simulink model "PSO_thuc_nghiem"  (R2021a)
settings: Solver=VariableStepAuto  StartTime=0.0  StopTime=10  RelTol=1e-3
InitFcn:
  | mc=0.5;
  | g=9.81;
  | n1=5;n2=1;
  | 
  | L2=0.5;
  | m1=2;
  | m2=mc;
  | m=5;
  | %Bo input shaping
  | alpha = (1/L1 + 1/L2)*(m1+m2)/m1;
  | beta = (((m1+m2)/m1)^2)*((1/L1 + 1/L2)^2) - 4*(m1+m2)/(m1*L1*L2);
  | w1 = sqrt(g*(alpha - sqrt(beta))/2);
  | w2 = sqrt(g*(alpha + sqrt(beta))/2);
  | damping_ratio = 0;
  | wd1 = w1*sqrt(1-damping_ratio^2);
  | wd2 = w2*sqrt(1-damping_ratio^2);
  | k = exp(damping_ratio*pi/sqrt(1-damping_ratio^2));
  | 
  | %ETM4_1
  | m_etm4_1 = 0.1;
  | I_etm4_1 = (1+m_etm4_1)*k*k/(k^2 + (1+m_etm4_1)*(k^(4/3)+k^(2/3)) + m_etm4_1);
  | A1_etm4_1 = I_etm4_1/(1+m_etm4_1);
  | A2_etm4_1 = I_etm4_1/(k^(2/3));
  | A3_etm4_1 = I_etm4_1/(k^(4/3));
  | A4_etm4_1 = m_etm4_1*I_etm4_1/((1+m_etm4_1)*(k^2));
  | t1_etm4_1 = (2*pi/3)/wd1;
  | t2_etm4_1 = (4*pi/3)/wd1;
  | t3_etm4_1 = 2*pi/wd1;
  | %ETM4_2
  | m_etm4_2 = 0.1;
  | I_etm4_2 = (1+m_etm4_2)*k*k/(k^2 + (1+m_etm4_2)*(k^(4/3)+k^(2/3)) + m_etm4_2);
  | A1_etm4_2 = I_etm4_2/(1+m_etm4_2);
  | A2_etm4_2 = I_etm4_2/(k^(2/3));
  | A3_etm4_2 = I_etm4_2/(k^(4/3));
  | A4_etm4_2 = m_etm4_2*I_etm4_2/((1+m_etm4_2)*(k^2));
  | t1_etm4_2 = (2*pi/3)/wd2;
  | t2_etm4_2 = (4*pi/3)/wd2;
  | t3_etm4_2 = 2*pi/wd2;
values from neighbouring files (symbols this model uses):
  l_ini = L    [PSO_ZVD.m]
  particle = repmat(empty_particle, nPop, 1)    [PSO16_12.m]    (also in PSO_ZVD.m)
undefined symbols (not defined in the file or in its folder): b0, b1, i, Kd, Kd1, Kp, Kp1, l, l1, l11, l2, l21, l3, l31, l_ref, li, M2, x_ref, xi
libraries: neural x70, simulink_extras x11, simulink x5
(part 21 of 25)

== matlab function PSO_thuc_nghiem/non linear model/con lắc đôi2/MATLAB Function ==
  data: z1 input; z2 input; z3 input; z4 input; z5 input; z6 input; z7 input; z8 input; d1z1 output; d1z2 output; d1z3 output; d1z4 output; d1z5 output; d1z6 output; d1z7 output; d1z8 output; ux input; ul input
function [d1z1,d1z2,d1z3,d1z4,d1z5,d1z6,d1z7,d1z8] = fcn(z1,z2, z3, z4, z5, z6, z7, z8, ux, ul)

m=20; m1=5; m2=1; l2= 0.2; g= 9.8;

d1z1=z2;
d1z2 =(m1*ul*sin(z5) - m2*ux - m1*ux + m2*ul*sin(z5) + m2*ux*cos(z5 - z7)^2 + m2*ux*sin(z5 - z7)^2 - m2*ul*sin(z5 - z7)*cos(z7) - g*m2^2*cos(z7)*sin(z7) - l2*m2^2*z8^2*sin(z7) - m2*ul*cos(z5 - z7)^2*sin(z5) + g*m2^2*cos(z5 - z7)*sin(z5 - z7)*cos(z5)^2 - g*m2^2*cos(z5 - z7)*sin(z5 - z7)*sin(z5)^2 + m2*ul*cos(z5 - z7)*sin(z5 - z7)*cos(z5) - g*m1*m2*cos(z7)*sin(z7) - l2*m1*m2*z8^2*sin(z7) + g*m2^2*cos(z5 - z7)*cos(z5)*sin(z7) + g*m2^2*cos(z5 - z7)*cos(z7)*sin(z5) - g*m2^2*sin(z5 - z7)*cos(z5)*cos(z7) + l2*m2^2*z8^2*cos(z5 - z7)*sin(z5) - l2*m2^2*z8^2*sin(z5 - z7)*cos(z5) + g*m2^2*sin(z5 - z7)*sin(z5)*sin(z7) - g*m2^2*cos(z5 - z7)^2*cos(z5)*sin(z5) - l2*m2^2*z8^2*cos(z5 - z7)^3*sin(z5) + l2*m2^2*z8^2*sin(z5 - z7)^3*cos(z5) + l2*m2^2*z8^2*cos(z5 - z7)^2*sin(z7) + g*m2^2*sin(z5 - z7)^2*cos(z5)*sin(z5) + l2*m2^2*z8^2*sin(z5 - z7)^2*sin(z7) + g*m1*m2*cos(z5 - z7)*sin(z5 - z7)*cos(z5)^2 - g*m1*m2*cos(z5 - z7)*sin(z5 - z7)*sin(z5)^2 + g*m1*m2*cos(z5 - z7)*cos(z5)*sin(z7) + g*m1*m2*cos(z5 - z7)*cos(z7)*sin(z5) - g*m1*m2*sin(z5 - z7)*cos(z5)*cos(z7) + l2*m1*m2*z8^2*cos(z5 - z7)*sin(z5) - l2*m1*m2*z8^2*sin(z5 - z7)*cos(z5) + g*m1*m2*sin(z5 - z7)*sin(z5)*sin(z7) - g*m1*m2*cos(z5 - z7)^2*cos(z5)*sin(z5) + l2*m2^2*z8^2*cos(z5 - z7)^2*sin(z5 - z7)*cos(z5) + g*m1*m2*sin(z5 - z7)^2*cos(z5)*sin(z5) - l2*m2^2*z8^2*cos(z5 - z7)*sin(z5 - z7)^2*sin(z5))/(m1^2*cos(z5)^2 - m*m2 - 2*m1*m2 - m*m1 + m2^2*cos(z5)^2 + m2^2*cos(z7)^2 + m1^2*sin(z5)^2 + m2^2*sin(z5)^2 + m2^2*cos(z5 - z7)^2 + m2^2*sin(z5 - z7)^2 - m1^2 - m2^2 + 2*m1*m2*cos(z5)^2 + m1*m2*cos(z7)^2 + 2*m1*m2*sin(z5)^2 + m*m2*cos(z5 - z7)^2 + m1*m2*cos(z5 - z7)^2 + m*m2*sin(z5 - z7)^2 + m1*m2*sin(z5 - z7)^2 - m2^2*cos(z5 - z7)^2*sin(z5)^2 - m2^2*sin(z5 - z7)^2*cos(z5)^2 - 2*m2^2*sin(z5 - z7)*cos(z7)*sin(z5) - m1*m2*cos(z5 - z7)^2*sin(z5)^2 - m1*m2*sin(z5 - z7)^2*cos(z5)^2 - 2*m2^2*cos(z5 - z7)*cos(z5)*cos(z7) - 2*m1*m2*cos(z5 - z7)*cos(z5)*cos(z7) - 2*m1*m2*sin(z5 - z7)*cos(z7)*sin(z5) + 2*m2^2*cos(z5 - z7)*sin(z5 - z7)*cos(z5)*sin(z5) + 2*m1*m2*cos(z5 - z7)*sin(z5 - z7)*cos(z5)*sin(z5));
d1z3=z4; 
d1z4 =(m2^2*ul*cos(z5 - z7)^2 - m2^2*ul - m1^2*ul - g*m1^3*cos(z5) - g*m2^3*cos(z5) - m1^3*z3*z6^2 - m2^3*z3*z6^2 + m1^2*ux*sin(z5) + m2^2*ux*sin(z5) - m*m1*ul - m*m2*ul - 2*m1*m2*ul + g*m1^3*cos(z5)^3 + g*m2^3*cos(z5)^3 + m1^2*ul*cos(z5)^2 + m2^2*ul*cos(z5)^2 + m2^2*ul*cos(z7)^2 - m2^2*ux*cos(z5 - z7)^2*sin(z5) + m2^3*z3*z6^2*sin(z5 - z7)^2 + m*m2*ul*cos(z5 - z7)^2 + m1*m2*ul*cos(z5 - z7)^2 + 3*g*m1*m2^2*cos(z5)^3 + 3*g*m1^2*m2*cos(z5)^3 - l2*m2^3*z8^2*cos(z5 - z7) + 2*m1*m2*ux*sin(z5) - m2^2*ux*sin(z5 - z7)*cos(z7) - g*m2^3*sin(z5 - z7)*sin(z7) + g*m2^3*cos(z5)*cos(z7)^2 + m1^3*z3*z6^2*cos(z5)^2 + m2^3*z3*z6^2*cos(z5)^2 + m2^3*z3*z6^2*cos(z7)^2 + g*m1^3*cos(z5)*sin(z5)^2 + g*m2^3*cos(z5)*sin(z5)^2 + m1^3*z3*z6^2*sin(z5)^2 + m2^3*z3*z6^2*sin(z5)^2 - g*m*m1^2*cos(z5) - g*m*m2^2*cos(z5) - 3*g*m1*m2^2*cos(z5) - 3*g*m1^2*m2*cos(z5) + g*m2^3*cos(z5 - z7)^2*cos(z5) + l2*m2^3*z8^2*cos(z5 - z7)^3 + 2*m1*m2*ul*cos(z5)^2 + m1*m2*ul*cos(z7)^2 - m*m1^2*z3*z6^2 - m*m2^2*z3*z6^2 - 3*m1*m2^2*z3*z6^2 - 3*m1^2*m2*z3*z6^2 + m2^3*z3*z6^2*cos(z5 - z7)^2 + l2*m2^3*z8^2*cos(z5 - z7)*sin(z5 - z7)^2 - m1*m2*ux*cos(z5 - z7)^2*sin(z5) - g*m*m2^2*sin(z5 - z7)*sin(z7) - 2*g*m1*m2^2*sin(z5 - z7)*sin(z7) - g*m1^2*m2*sin(z5 - z7)*sin(z7) + 2*g*m1*m2^2*cos(z5)*cos(z7)^2 + g*m1^2*m2*cos(z5)*cos(z7)^2 + 3*m1*m2^2*z3*z6^2*cos(z5)^2 + 3*m1^2*m2*z3*z6^2*cos(z5)^2 + 2*m1*m2^2*z3*z6^2*cos(z7)^2 + m1^2*m2*z3*z6^2*cos(z7)^2 + 3*g*m1*m2^2*cos(z5)*sin(z5)^2 + 3*g*m1^2*m2*cos(z5)*sin(z5)^2 + 3*m1*m2^2*z3*z6^2*sin(z5)^2 + 3*m1^2*m2*z3*z6^2*sin(z5)^2 - m2^3*z3*z6^2*cos(z5 - z7)^2*sin(z5)^2 - m2^3*z3*z6^2*sin(z5 - z7)^2*cos(z5)^2 + g*m2^3*cos(z7)*sin(z5)*sin(z7) + l2*m2^3*z8^2*sin(z5)*sin(z7) + g*m*m2^2*cos(z5 - z7)^2*cos(z5) + 2*g*m1*m2^2*cos(z5 - z7)^2*cos(z5) + g*m1^2*m2*cos(z5 - z7)^2*cos(z5) + l2*m*m2^2*z8^2*cos(z5 - z7)^3 + l2*m1*m2^2*z8^2*cos(z5 - z7)^3 + m*m2^2*z3*z6^2*cos(z5 - z7)^2 + 2*m1*m2^2*z3*z6^2*cos(z5 - z7)^2 + m1^2*m2*z3*z6^2*cos(z5 - z7)^2 + m*m2^2*z3*z6^2*sin(z5 - z7)^2 + 2*m1*m2^2*z3*z6^2*sin(z5 - z7)^2 + m1^2*m2*z3*z6^2*sin(z5 - z7)^2 - 2*m2^2*ul*cos(z5 - z7)*cos(z5)*cos(z7) - m1*m2*ux*sin(z5 - z7)*cos(z7) + m2^2*ux*cos(z5 - z7)*sin(z5 - z7)*cos(z5) + g*m2^3*cos(z5 - z7)*sin(z5 - z7)*sin(z5) - 2*g*m2^3*cos(z5 - z7)*cos(z5)^2*cos(z7) + l2*m2^3*z8^2*cos(z5 - z7)*cos(z5)^2 + l2*m2^3*z8^2*cos(z5 - z7)*cos(z7)^2 - g*m2^3*cos(z5 - z7)*cos(z7)*sin(z5)^2 + g*m2^3*sin(z5 - z7)*cos(z5)^2*sin(z7) - 2*g*m*m1*m2*cos(z5) - l2*m*m2^2*z8^2*cos(z5 - z7) - 2*l2*m1*m2^2*z8^2*cos(z5 - z7) - l2*m1^2*m2*z8^2*cos(z5 - z7) - 2*m*m1*m2*z3*z6^2 - l2*m*m1*m2*z8^2*cos(z5 - z7) - g*m*m1*m2*sin(z5 - z7)*sin(z7) + g*m*m2^2*cos(z5 - z7)*sin(z5 - z7)*sin(z5) + 2*g*m1*m2^2*cos(z5 - z7)*sin(z5 - z7)*sin(z5) + g*m1^2*m2*cos(z5 - z7)*sin(z5 - z7)*sin(z5) - 4*g*m1*m2^2*cos(z5 - z7)*cos(z5)^2*cos(z7) - 2*g*m1^2*m2*cos(z5 - z7)*cos(z5)^2*cos(z7) + 2*l2*m1*m2^2*z8^2*cos(z5 - z7)*cos(z5)^2 + l2*m1^2*m2*z8^2*cos(z5 - z7)*cos(z5)^2 + l2*m1*m2^2*z8^2*cos(z5 - z7)*cos(z7)^2 - 2*g*m1*m2^2*cos(z5 - z7)*cos(z7)*sin(z5)^2 - g*m1^2*m2*cos(z5 - z7)*cos(z7)*sin(z5)^2 + 2*g*m1*m2^2*sin(z5 - z7)*cos(z5)^2*sin(z7) + g*m1^2*m2*sin(z5 - z7)*cos(z5)^2*sin(z7) - 2*m2^3*z3*z6^2*cos(z5 - z7)*cos(z5)*cos(z7) + g*m*m1*m2*cos(z5 - z7)^2*cos(z5) - g*m2^3*cos(z5 - z7)*cos(z5)*sin(z5)*sin(z7) - g*m2^3*sin(z5 - z7)*cos(z5)*cos(z7)*sin(z5) + l2*m2^3*z8^2*sin(z5 - z7)*cos(z5)*sin(z5) - l2*m2^3*z8^2*sin(z5 - z7)*cos(z7)*sin(z7) + m*m1*m2*z3*z6^2*cos(z5 - z7)^2 - 2*m2^3*z3*z6^2*sin(z5 - z7)*cos(z7)*sin(z5) + l2*m*m2^2*z8^2*cos(z5 - z7)*sin(z5 - z7)^2 + l2*m1*m2^2*z8^2*cos(z5 - z7)*sin(z5 - z7)^2 + m*m1*m2*z3*z6^2*sin(z5 - z7)^2 - 2*m1*m2*ul*cos(z5 - z7)*cos(z5)*cos(z7) - 2*l2*m2^3*z8^2*cos(z5 - z7)^2*cos(z5)*cos(z7) - 2*m1*m2^2*z3*z6^2*cos(z5 - z7)^2*sin(z5)^2 - 2*m1*m2^2*z3*z6^2*sin(z5 - z7)^2*cos(z5)^2 - m1^2*m2*z3*z6^2*cos(z5 - z7)^2*sin(z5)^2 - m1^2*m2*z3*z6^2*sin(z5 - z7)^2*cos(z5)^2 - l2*m2^3*z8^2*sin(z5 - z7)^2*cos(z5)*cos(z7) + 2*g*m1*m2^2*cos(z7)*sin(z5)*sin(z7) + g*m1^2*m2*cos(z7)*sin(z5)*sin(z7) + 2*l2*m1*m2^2*z8^2*sin(z5)*sin(z7) + l2*m1^2*m2*z8^2*sin(z5)*sin(z7) - l2*m2^3*z8^2*cos(z5 - z7)^2*sin(z5)*sin(z7) + m1*m2*ux*cos(z5 - z7)*sin(z5 - z7)*cos(z5) - 2*l2*m1*m2^2*z8^2*cos(z5 - z7)^2*cos(z5)*cos(z7) - l2*m1*m2^2*z8^2*sin(z5 - z7)^2*cos(z5)*cos(z7) - l2*m1*m2^2*z8^2*cos(z5 - z7)^2*sin(z5)*sin(z7) + g*m*m1*m2*cos(z5 - z7)*sin(z5 - z7)*sin(z5) + l2*m2^3*z8^2*cos(z5 - z7)*sin(z5 - z7)*cos(z5)*sin(z7) - l2*m2^3*z8^2*cos(z5 - z7)*sin(z5 - z7)*cos(z7)*sin(z5) + 2*m2^3*z3*z6^2*cos(z5 - z7)*sin(z5 - z7)*cos(z5)*sin(z5) - 4*m1*m2^2*z3*z6^2*cos(z5 - z7)*cos(z5)*cos(z7) - 2*m1^2*m2*z3*z6^2*cos(z5 - z7)*cos(z5)*cos(z7) - 2*g*m1*m2^2*cos(z5 - z7)*cos(z5)*sin(z5)*sin(z7) - 2*g*m1*m2^2*sin(z5 - z7)*cos(z5)*cos(z7)*sin(z5) - g*m1^2*m2*cos(z5 - z7)*cos(z5)*sin(z5)*sin(z7) - g*m1^2*m2*sin(z5 - z7)*cos(z5)*cos(z7)*sin(z5) + 2*l2*m1*m2^2*z8^2*sin(z5 - z7)*cos(z5)*sin(z5) + l2*m1^2*m2*z8^2*sin(z5 - z7)*cos(z5)*sin(z5) - l2*m1*m2^2*z8^2*sin(z5 - z7)*cos(z7)*sin(z7) - 4*m1*m2^2*z3*z6^2*sin(z5 - z7)*cos(z7)*sin(z5) - 2*m1^2*m2*z3*z6^2*sin(z5 - z7)*cos(z7)*sin(z5) + l2*m1*m2^2*z8^2*cos(z5 - z7)*sin(z5 - z7)*cos(z5)*sin(z7) - l2*m1*m2^2*z8^2*cos(z5 - z7)*sin(z5 - z7)*cos(z7)*sin(z5) + 4*m1*m2^2*z3*z6^2*cos(z5 - z7)*sin(z5 - z7)*cos(z5)*sin(z5) + 2*m1^2*m2*z3*z6^2*cos(z5 - z7)*sin(z5 - z7)*cos(z5)*sin(z5))/((m1 + m2)*(m1^2*cos(z5)^2 - m*m2 - 2*m1*m2 - m*m1 + m2^2*cos(z5)^2 + m2^2*cos(z7)^2 + m1^2*sin(z5)^2 + m2^2*sin(z5)^2 + m2^2*cos(z5 - z7)^2 + m2^2*sin(z5 - z7)^2 - m1^2 - m2^2 + 2*m1*m2*cos(z5)^2 + m1*m2*cos(z7)^2 + 2*m1*m2*sin(z5)^2 + m*m2*cos(z5 - z7)^2 + m1*m2*cos(z5 - z7)^2 + m*m2*sin(z5 - z7)^2 + m1*m2*sin(z5 - z7)^2 - m2^2*cos(z5 - z7)^2*sin(z5)^2 - m2^2*sin(z5 - z7)^2*cos(z5)^2 - 2*m2^2*sin(z5 - z7)*cos(z7)*sin(z5) - m1*m2*cos(z5 - z7)^2*sin(z5)^2 - m1*m2*sin(z5 - z7)^2*cos(z5)^2 - 2*m2^2*cos(z5 - z7)*cos(z5)*cos(z7) - 2*m1*m2*cos(z5 - z7)*cos(z5)*cos(z7) - 2*m1*m2*sin(z5 - z7)*cos(z7)*sin(z5) + 2*m2^2*cos(z5 - z7)*sin(z5 - z7)*cos(z5)*sin(z5) + 2*m1*m2*cos(z5 - z7)*sin(z5 - z7)*cos(z5)*sin(z5)));
d1z5=z6; 
d1z6 =-(g*m1^3*sin(z5)^3 - 2*m2^3*z4*z6 - m1^2*ux*cos(z5) - m2^2*ux*cos(z5) - g*m1^3*sin(z5) - g*m2^3*sin(z5) - 2*m1^3*z4*z6 + g*m2^3*sin(z5)^3 + m2^2*ux*sin(z5 - z7)^2*cos(z5) + g*m2^3*sin(z5 - z7)^2*sin(z5) + 3*g*m1*m2^2*sin(z5)^3 + 3*g*m1^2*m2*sin(z5)^3 + 2*m1^3*z4*z6*cos(z5)^2 + 2*m2^3*z4*z6*cos(z5)^2 + 2*m2^3*z4*z6*cos(z7)^2 + m1^2*ul*cos(z5)*sin(z5) + m2^2*ul*cos(z5)*sin(z5) + 2*m1^3*z4*z6*sin(z5)^2 + 2*m2^3*z4*z6*sin(z5)^2 - 2*m1*m2*ux*cos(z5) - 2*m*m1^2*z4*z6 - 2*m*m2^2*z4*z6 - 6*m1*m2^2*z4*z6 - 6*m1^2*m2*z4*z6 + m2^2*ux*cos(z5 - z7)*cos(z7) + 2*m2^3*z4*z6*cos(z5 - z7)^2 + g*m2^3*cos(z5 - z7)*sin(z7) - l2*m2^3*z8^2*sin(z5 - z7) + 2*m2^3*z4*z6*sin(z5 - z7)^2 + g*m1^3*cos(z5)^2*sin(z5) + g*m2^3*cos(z5)^2*sin(z5) + g*m2^3*cos(z7)^2*sin(z5) + m2^2*ul*cos(z5 - z7)*sin(z5 - z7) - g*m*m1^2*sin(z5) - g*m*m2^2*sin(z5) - 3*g*m1*m2^2*sin(z5) - 3*g*m1^2*m2*sin(z5) + l2*m2^3*z8^2*sin(z5 - z7)^3 + 2*m*m2^2*z4*z6*cos(z5 - z7)^2 + 4*m1*m2^2*z4*z6*cos(z5 - z7)^2 + 2*m1^2*m2*z4*z6*cos(z5 - z7)^2 + g*m*m2^2*cos(z5 - z7)*sin(z7) + 2*g*m1*m2^2*cos(z5 - z7)*sin(z7) + g*m1^2*m2*cos(z5 - z7)*sin(z7) - l2*m*m2^2*z8^2*sin(z5 - z7) - 2*l2*m1*m2^2*z8^2*sin(z5 - z7) - l2*m1^2*m2*z8^2*sin(z5 - z7) + l2*m2^3*z8^2*cos(z5 - z7)^2*sin(z5 - z7) + m1*m2*ux*sin(z5 - z7)^2*cos(z5) + 2*m*m2^2*z4*z6*sin(z5 - z7)^2 + 4*m1*m2^2*z4*z6*sin(z5 - z7)^2 + 2*m1^2*m2*z4*z6*sin(z5 - z7)^2 + 3*g*m1*m2^2*cos(z5)^2*sin(z5) + 3*g*m1^2*m2*cos(z5)^2*sin(z5) + 2*g*m1*m2^2*cos(z7)^2*sin(z5) + g*m1^2*m2*cos(z7)^2*sin(z5) - g*m2^3*cos(z5)*cos(z7)*sin(z7) - l2*m2^3*z8^2*cos(z5)*sin(z7) + l2*m*m2^2*z8^2*sin(z5 - z7)^3 + l2*m1*m2^2*z8^2*sin(z5 - z7)^3 + g*m*m2^2*sin(z5 - z7)^2*sin(z5) + 2*g*m1*m2^2*sin(z5 - z7)^2*sin(z5) + g*m1^2*m2*sin(z5 - z7)^2*sin(z5) + 2*m1*m2*ul*cos(z5)*sin(z5) - m2^2*ul*cos(z5 - z7)*cos(z7)*sin(z5) - m2^2*ul*sin(z5 - z7)*cos(z5)*cos(z7) - 4*m*m1*m2*z4*z6 + m1*m2*ux*cos(z5 - z7)*cos(z7) + g*m2^3*cos(z5 - z7)*sin(z5 - z7)*cos(z5) + 6*m1*m2^2*z4*z6*cos(z5)^2 + 6*m1^2*m2*z4*z6*cos(z5)^2 + 4*m1*m2^2*z4*z6*cos(z7)^2 + 2*m1^2*m2*z4*z6*cos(z7)^2 - m2^2*ux*cos(z5 - z7)*sin(z5 - z7)*sin(z5) - g*m2^3*sin(z5 - z7)*cos(z5)^2*cos(z7) + l2*m2^3*z8^2*sin(z5 - z7)*cos(z7)^2 + 6*m1*m2^2*z4*z6*sin(z5)^2 + 6*m1^2*m2*z4*z6*sin(z5)^2 - 2*m2^3*z4*z6*cos(z5 - z7)^2*sin(z5)^2 - 2*m2^3*z4*z6*sin(z5 - z7)^2*cos(z5)^2 - g*m2^3*cos(z5 - z7)*sin(z5)^2*sin(z7) - 2*g*m2^3*sin(z5 - z7)*cos(z7)*sin(z5)^2 + l2*m2^3*z8^2*sin(z5 - z7)*sin(z5)^2 + m*m2*ul*cos(z5 - z7)*sin(z5 - z7) + m1*m2*ul*cos(z5 - z7)*sin(z5 - z7) - 2*g*m*m1*m2*sin(z5) + 2*m*m1*m2*z4*z6*cos(z5 - z7)^2 - 4*m2^3*z4*z6*sin(z5 - z7)*cos(z7)*sin(z5) + g*m*m1*m2*cos(z5 - z7)*sin(z7) - l2*m*m1*m2*z8^2*sin(z5 - z7) + g*m*m2^2*cos(z5 - z7)*sin(z5 - z7)*cos(z5) + 2*g*m1*m2^2*cos(z5 - z7)*sin(z5 - z7)*cos(z5) + g*m1^2*m2*cos(z5 - z7)*sin(z5 - z7)*cos(z5) + 2*m*m1*m2*z4*z6*sin(z5 - z7)^2 - 2*g*m1*m2^2*sin(z5 - z7)*cos(z5)^2*cos(z7) - g*m1^2*m2*sin(z5 - z7)*cos(z5)^2*cos(z7) + l2*m1*m2^2*z8^2*sin(z5 - z7)*cos(z7)^2 - 4*m1*m2^2*z4*z6*cos(z5 - z7)^2*sin(z5)^2 - 4*m1*m2^2*z4*z6*sin(z5 - z7)^2*cos(z5)^2 - 2*m1^2*m2*z4*z6*cos(z5 - z7)^2*sin(z5)^2 - 2*m1^2*m2*z4*z6*sin(z5 - z7)^2*cos(z5)^2 - 2*g*m1*m2^2*cos(z5 - z7)*sin(z5)^2*sin(z7) - 4*g*m1*m2^2*sin(z5 - z7)*cos(z7)*sin(z5)^2 - g*m1^2*m2*cos(z5 - z7)*sin(z5)^2*sin(z7) - 2*g*m1^2*m2*sin(z5 - z7)*cos(z7)*sin(z5)^2 + 2*l2*m1*m2^2*z8^2*sin(z5 - z7)*sin(z5)^2 + l2*m1^2*m2*z8^2*sin(z5 - z7)*sin(z5)^2 - g*m2^3*cos(z5 - z7)*cos(z5)*cos(z7)*sin(z5) + l2*m2^3*z8^2*cos(z5 - z7)*cos(z5)*sin(z5) + l2*m2^3*z8^2*cos(z5 - z7)*cos(z7)*sin(z7) + g*m2^3*sin(z5 - z7)*cos(z5)*sin(z5)*sin(z7) + l2*m*m2^2*z8^2*cos(z5 - z7)^2*sin(z5 - z7) + l2*m1*m2^2*z8^2*cos(z5 - z7)^2*sin(z5 - z7) + g*m*m1*m2*sin(z5 - z7)^2*sin(z5) - m1*m2*ul*cos(z5 - z7)*cos(z7)*sin(z5) - m1*m2*ul*sin(z5 - z7)*cos(z5)*cos(z7) - 2*g*m1*m2^2*cos(z5)*cos(z7)*sin(z7) - g*m1^2*m2*cos(z5)*cos(z7)*sin(z7) - 2*l2*m1*m2^2*z8^2*cos(z5)*sin(z7) - l2*m1^2*m2*z8^2*cos(z5)*sin(z7) - l2*m2^3*z8^2*cos(z5 - z7)^2*cos(z7)*sin(z5) + l2*m2^3*z8^2*sin(z5 - z7)^2*cos(z5)*sin(z7) - 2*l2*m2^3*z8^2*sin(z5 - z7)^2*cos(z7)*sin(z5) - m1*m2*ux*cos(z5 - z7)*sin(z5 - z7)*sin(z5) - 4*m2^3*z4*z6*cos(z5 - z7)*cos(z5)*cos(z7) - l2*m1*m2^2*z8^2*cos(z5 - z7)^2*cos(z7)*sin(z5) + 4*m2^3*z4*z6*cos(z5 - z7)*sin(z5 - z7)*cos(z5)*sin(z5) + g*m*m1*m2*cos(z5 - z7)*sin(z5 - z7)*cos(z5) + l2*m1*m2^2*z8^2*sin(z5 - z7)^2*cos(z5)*sin(z7) - 2*l2*m1*m2^2*z8^2*sin(z5 - z7)^2*cos(z7)*sin(z5) - 8*m1*m2^2*z4*z6*cos(z5 - z7)*cos(z5)*cos(z7) - 4*m1^2*m2*z4*z6*cos(z5 - z7)*cos(z5)*cos(z7) - l2*m2^3*z8^2*cos(z5 - z7)*sin(z5 - z7)*cos(z5)*cos(z7) - 8*m1*m2^2*z4*z6*sin(z5 - z7)*cos(z7)*sin(z5) - 4*m1^2*m2*z4*z6*sin(z5 - z7)*cos(z7)*sin(z5) - l2*m2^3*z8^2*cos(z5 - z7)*sin(z5 - z7)*sin(z5)*sin(z7) - 2*g*m1*m2^2*cos(z5 - z7)*cos(z5)*cos(z7)*sin(z5) - g*m1^2*m2*cos(z5 - z7)*cos(z5)*cos(z7)*sin(z5) + 2*l2*m1*m2^2*z8^2*cos(z5 - z7)*cos(z5)*sin(z5) + l2*m1^2*m2*z8^2*cos(z5 - z7)*cos(z5)*sin(z5) + l2*m1*m2^2*z8^2*cos(z5 - z7)*cos(z7)*sin(z7) + 2*g*m1*m2^2*sin(z5 - z7)*cos(z5)*sin(z5)*sin(z7) + g*m1^2*m2*sin(z5 - z7)*cos(z5)*sin(z5)*sin(z7) + 8*m1*m2^2*z4*z6*cos(z5 - z7)*sin(z5 - z7)*cos(z5)*sin(z5) + 4*m1^2*m2*z4*z6*cos(z5 - z7)*sin(z5 - z7)*cos(z5)*sin(z5) - l2*m1*m2^2*z8^2*cos(z5 - z7)*sin(z5 - z7)*cos(z5)*cos(z7) - l2*m1*m2^2*z8^2*cos(z5 - z7)*sin(z5 - z7)*sin(z5)*sin(z7))/(z3*(m1 + m2)*(m1^2*cos(z5)^2 - m*m2 - 2*m1*m2 - m*m1 + m2^2*cos(z5)^2 + m2^2*cos(z7)^2 + m1^2*sin(z5)^2 + m2^2*sin(z5)^2 + m2^2*cos(z5 - z7)^2 + m2^2*sin(z5 - z7)^2 - m1^2 - m2^2 + 2*m1*m2*cos(z5)^2 + m1*m2*cos(z7)^2 + 2*m1*m2*sin(z5)^2 + m*m2*cos(z5 - z7)^2 + m1*m2*cos(z5 - z7)^2 + m*m2*sin(z5 - z7)^2 + m1*m2*sin(z5 - z7)^2 - m2^2*cos(z5 - z7)^2*sin(z5)^2 - m2^2*sin(z5 - z7)^2*cos(z5)^2 - 2*m2^2*sin(z5 - z7)*cos(z7)*sin(z5) - m1*m2*cos(z5 - z7)^2*sin(z5)^2 - m1*m2*sin(z5 - z7)^2*cos(z5)^2 - 2*m2^2*cos(z5 - z7)*cos(z5)*cos(z7) - 2*m1*m2*cos(z5 - z7)*cos(z5)*cos(z7) - 2*m1*m2*sin(z5 - z7)*cos(z7)*sin(z5) + 2*m2^2*cos(z5 - z7)*sin(z5 - z7)*cos(z5)*sin(z5) + 2*m1*m2*cos(z5 - z7)*sin(z5 - z7)*cos(z5)*sin(z5)));
d1z7 = z8;
d1z8 =-(m1*ul*cos(z7)*sin(z5) - m2*ux*cos(z7) - m*ul*sin(z5 - z7) - m1*ul*sin(z5 - z7) - m2*ul*sin(z5 - z7) - g*m1^2*sin(z7) - g*m2^2*sin(z7) - m1*ux*cos(z7) + m2*ul*cos(z7)*sin(z5) + m1*ux*cos(z5 - z7)*cos(z5) + m2*ux*cos(z5 - z7)*cos(z5) + m1*ux*sin(z5 - z7)*sin(z5) + m2*ux*sin(z5 - z7)*sin(z5) - g*m*m1*sin(z7) - g*m*m2*sin(z7) - 2*g*m1*m2*sin(z7) + g*m1^2*cos(z5 - z7)*sin(z5) - g*m1^2*sin(z5 - z7)*cos(z5) + g*m2^2*cos(z5 - z7)*sin(z5) - g*m2^2*sin(z5 - z7)*cos(z5) + m1*ul*sin(z5 - z7)*cos(z5)^2 + m2*ul*sin(z5 - z7)*cos(z5)^2 + g*m1^2*cos(z5)^2*sin(z7) + g*m2^2*cos(z5)^2*sin(z7) + g*m1^2*sin(z5)^2*sin(z7) + g*m2^2*sin(z5)^2*sin(z7) - g*m1^2*cos(z5 - z7)*sin(z5)^3 + g*m1^2*sin(z5 - z7)*cos(z5)^3 - g*m2^2*cos(z5 - z7)*sin(z5)^3 + g*m2^2*sin(z5 - z7)*cos(z5)^3 - 2*g*m1*m2*cos(z5 - z7)*sin(z5)^3 + 2*g*m1*m2*sin(z5 - z7)*cos(z5)^3 - m1*ul*cos(z5 - z7)*cos(z5)*sin(z5) - m2*ul*cos(z5 - z7)*cos(z5)*sin(z5) - l2*m2^2*z8^2*cos(z7)*sin(z7) + g*m*m1*cos(z5 - z7)*sin(z5) - g*m*m1*sin(z5 - z7)*cos(z5) + g*m*m2*cos(z5 - z7)*sin(z5) - g*m*m2*sin(z5 - z7)*cos(z5) + 2*g*m1*m2*cos(z5 - z7)*sin(z5) - 2*g*m1*m2*sin(z5 - z7)*cos(z5) + 2*g*m1*m2*cos(z5)^2*sin(z7) - g*m1^2*cos(z5 - z7)*cos(z5)^2*sin(z5) - g*m2^2*cos(z5 - z7)*cos(z5)^2*sin(z5) + 2*g*m1*m2*sin(z5)^2*sin(z7) + g*m1^2*sin(z5 - z7)*cos(z5)*sin(z5)^2 + g*m2^2*sin(z5 - z7)*cos(z5)*sin(z5)^2 - l2*m1*m2*z8^2*cos(z7)*sin(z7) + l2*m2^2*z8^2*cos(z5 - z7)*cos(z5)*sin(z7) + l2*m2^2*z8^2*cos(z5 - z7)*cos(z7)*sin(z5) - l2*m2^2*z8^2*sin(z5 - z7)*cos(z5)*cos(z7) + l2*m2^2*z8^2*sin(z5 - z7)*sin(z5)*sin(z7) - l2*m2^2*z8^2*cos(z5 - z7)^2*cos(z5)*sin(z5) + l2*m2^2*z8^2*sin(z5 - z7)^2*cos(z5)*sin(z5) - 2*g*m1*m2*cos(z5 - z7)*cos(z5)^2*sin(z5) + l2*m2^2*z8^2*cos(z5 - z7)*sin(z5 - z7)*cos(z5)^2 + 2*g*m1*m2*sin(z5 - z7)*cos(z5)*sin(z5)^2 - l2*m2^2*z8^2*cos(z5 - z7)*sin(z5 - z7)*sin(z5)^2 - l2*m1*m2*z8^2*cos(z5 - z7)*sin(z5 - z7)*sin(z5)^2 + l2*m1*m2*z8^2*cos(z5 - z7)*cos(z5)*sin(z7) + l2*m1*m2*z8^2*cos(z5 - z7)*cos(z7)*sin(z5) - l2*m1*m2*z8^2*sin(z5 - z7)*cos(z5)*cos(z7) + l2*m1*m2*z8^2*sin(z5 - z7)*sin(z5)*sin(z7) - l2*m1*m2*z8^2*cos(z5 - z7)^2*cos(z5)*sin(z5) + l2*m1*m2*z8^2*sin(z5 - z7)^2*cos(z5)*sin(z5) + l2*m1*m2*z8^2*cos(z5 - z7)*sin(z5 - z7)*cos(z5)^2)/(l2*(m1^2*cos(z5)^2 - m*m2 - 2*m1*m2 - m*m1 + m2^2*cos(z5)^2 + m2^2*cos(z7)^2 + m1^2*sin(z5)^2 + m2^2*sin(z5)^2 + m2^2*cos(z5 - z7)^2 + m2^2*sin(z5 - z7)^2 - m1^2 - m2^2 + 2*m1*m2*cos(z5)^2 + m1*m2*cos(z7)^2 + 2*m1*m2*sin(z5)^2 + m*m2*cos(z5 - z7)^2 + m1*m2*cos(z5 - z7)^2 + m*m2*sin(z5 - z7)^2 + m1*m2*sin(z5 - z7)^2 - m2^2*cos(z5 - z7)^2*sin(z5)^2 - m2^2*sin(z5 - z7)^2*cos(z5)^2 - 2*m2^2*sin(z5 - z7)*cos(z7)*sin(z5) - m1*m2*cos(z5 - z7)^2*sin(z5)^2 - m1*m2*sin(z5 - z7)^2*cos(z5)^2 - 2*m2^2*cos(z5 - z7)*cos(z5)*cos(z7) - 2*m1*m2*cos(z5 - z7)*cos(z5)*cos(z7) - 2*m1*m2*sin(z5 - z7)*cos(z7)*sin(z5) + 2*m2^2*cos(z5 - z7)*sin(z5 - z7)*cos(z5)*sin(z5) + 2*m1*m2*cos(z5 - z7)*sin(z5 - z7)*cos(z5)*sin(z5)));

== matlab function PSO_thuc_nghiem/Hieu/Model_3/Crane ==
  data: x1 input; dx1 output; x2 input; x3 input; x4 input; x5 input; x6 input; ut input; ul input; dx2 output; dx3 output; dx4 output; dx5 output; dx6 output
function [dx1,dx2,dx3,dx4,dx5,dx6] = fcn(x1,x2,x3,x4,x5,x6,ut,ul)
mc = 0.85; mt =5; ml =2; bt =20; br =50; g =9.81;

dx1 = x2;
dx2 = -(bt*x2 *mc - ml*ut - mc*ul*sin(x5) - mc*ut + bt*x2 *ml ...
- x6^2*x3*mc^2*sin(x5) + br*x4*mc*sin(x5) + x6^2*x3*mc*ml*sin(x5) ...
+ g*mc*ml*cos(x5)*sin(x5))/(mc*ml + mc*mt + ml*mt - mc^2*cos(x5)^2 ...
- mc^2*sin(x5)^2 + mc^2 - mc*ml*cos(x5)^2);
% -(bt*d1x*mc - ml*ut - mc*ul*sin(the) - mc*ut + bt*d1x*ml 
% - d1the^2*l*mc^2*sin(the) + br*d1l*mc*sin(the) + d1the^2*l*mc*ml*sin(the) 
% + g*mc*ml*cos(the)*sin(the))/(mc*ml + mc*mt + ml*mt - mc^2*cos(the)^2 
% - mc^2*sin(the)^2 + mc^2 - mc*ml*cos(the)^2)

dx3 = x4;
dx4 = (mc*ul + mt*ul + mc*ut*sin(x5) + 2*x6^2*x3*mc^2 + g*mc^2*cos(x5) ...
- mc*ul*cos(x5)^2 - br*x4*mc - br*x4*mt - g*mc^2*cos(x5)^3 + 2*x6^2*x3*mc*mt ...
+ g*mc*mt*cos(x5) - bt*x2 *mc*sin(x5) - 2*x6^2*x3*mc^2*cos(x5)^2  ...
- x6^2*x3*mc^2*sin(x5)^2 - g*mc^2*cos(x5)*sin(x5)^2 ...
+ br*x4*mc*cos(x5)^2)/(mc*ml + mc*mt + ml*mt - mc^2*cos(x5)^2 ...
- mc^2*sin(x5)^2 + mc^2 - mc*ml*cos(x5)^2);
% (mc*ul + mt*ul + mc*ut*sin(the) + 2*d1the^2*l*mc^2 + g*mc^2*cos(the)
% - mc*ul*cos(the)^2 - br*d1l*mc - br*d1l*mt - g*mc^2*cos(the)^3 + 2*d1the^2*l*mc*mt 
% + g*mc*mt*cos(the) - bt*d1x*mc*sin(the) - 2*d1the^2*l*mc^2*cos(the)^2 
% - d1the^2*l*mc^2*sin(the)^2 - g*mc^2*cos(the)*sin(the)^2 
% + br*d1l*mc*cos(the)^2)/(mc*ml + mc*mt + ml*mt - mc^2*cos(the)^2 
% - mc^2*sin(the)^2 + mc^2 - mc*ml*cos(the)^2)

dx5 = x6;
dx6 = -(g*mc^2*sin(x5) - ml*ut*cos(x5) - mc*ut*cos(x5) - g*mc^2*sin(x5)^3 ...
+ 2*x4*x6*mc^2 - mc*ul*cos(x5)*sin(x5) + 2*x4*x6*mc*ml ...
+ 2*x4*x6*mc*mt + 2*x4*x6*ml*mt - 2*x4*x6*mc^2*cos(x5)^2 ...
- 2*x4*x6*mc^2*sin(x5)^2 + bt*x2 *mc*cos(x5) + bt*x2 *ml*cos(x5)...
+ g*mc*ml*sin(x5) + g*mc*mt*sin(x5) + g*ml*mt*sin(x5) ...
- g*mc^2*cos(x5)^2*sin(x5) - x6^2*x3*mc^2*cos(x5)*sin(x5) ...
- 2*x4*x6*mc*ml*cos(x5)^2 + br*x4*mc*cos(x5)*sin(x5) ...
+ x6^2*x3*mc*ml*cos(x5)*sin(x5))/(x3*(mc*ml + mc*mt + ml*mt ...
- mc^2*cos(x5)^2 - mc^2*sin(x5)^2 + mc^2 - mc*ml*cos(x5)^2));
% -(g*mc^2*sin(the) - ml*ut*cos(the) - mc*ut*cos(the) - g*mc^2*sin(the)^3 
% + 2*d1l*d1the*mc^2 - mc*ul*cos(the)*sin(the) + 2*d1l*d1the*mc*ml 
% + 2*d1l*d1the*mc*mt + 2*d1l*d1the*ml*mt - 2*d1l*d1the*mc^2*cos(the)^2 
% - 2*d1l*d1the*mc^2*sin(the)^2 + bt*d1x*mc*cos(the) + bt*d1x*ml*cos(the) 
% + g*mc*ml*sin(the) + g*mc*mt*sin(the) + g*ml*mt*sin(the) 
% - g*mc^2*cos(the)^2*sin(the) - d1the^2*l*mc^2*cos(the)*sin(the) 
% - 2*d1l*d1the*mc*ml*cos(the)^2 + br*d1l*mc*cos(the)*sin(the) 
% + d1the^2*l*mc*ml*cos(the)*sin(the))/(l*(mc*ml + mc*mt + ml*mt 
% - mc^2*cos(the)^2 - mc^2*sin(the)^2 + mc^2 - mc*ml*cos(the)^2))
